simulink model "TMPC_3"  (Simulink 9.1)
settings: Solver=ode45  StartTime=0.0  StopTime=6  FixedStep=0.01  RelTol=1e-3  EnableMultiTasking=on
undefined symbols (not defined in the file): random_seeds
libraries: simulink x4, Solver_SF x1
settings Model: Creator=xuwei  LastModifiedBy=CK12
settings DataIOCC: LimitDataPoints=on
settings OptimizationCC: ExpressionDepthLimit=2147483647
settings DebuggingCC: SolverPrmCheckMsg=warning  FcnCallInpInsideContextMsg=warning  StateNameClashWarn=warning
settings ConfigComp: CovHtmlReporting=off

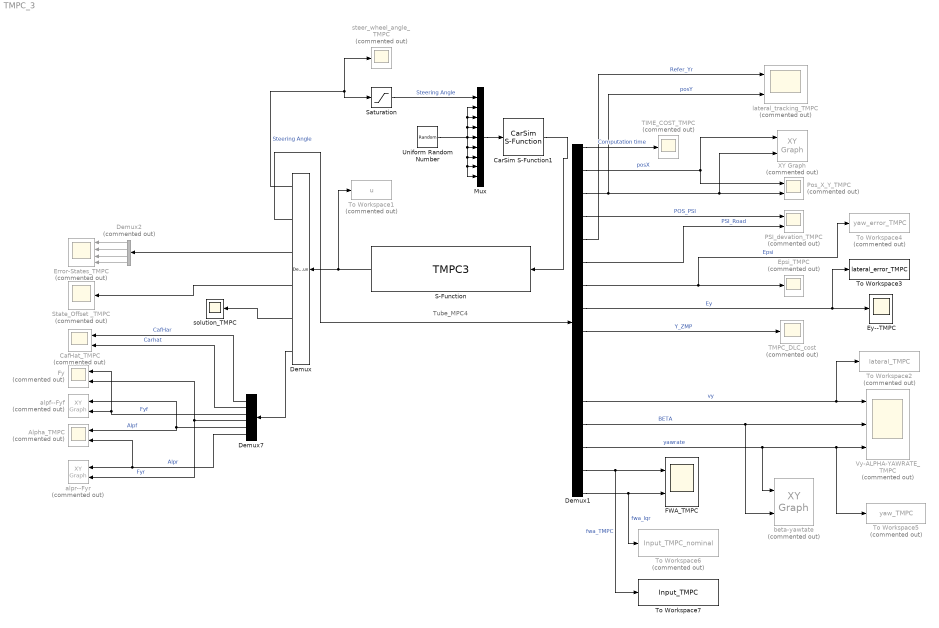
== system TMPC_3 ==
  note: Tube_MPC4
  Alpha_TMPC : Scope  Commented=on  NumInputPorts=2
  CafHat_TMPC : Scope  Commented=on  NumInputPorts=2
  CarSim S-Function1 : Solver_SF/CarSim S-Function  Priority=1  SIMFILE=simfile.sim  Run_RTs=off  vs_state_ind=Run  StopMode_ind=Vehicle Model
  Demux : Demux  Outputs=[1 16 4 4 1 6]
  Demux1 : Demux  Outputs=16
  Demux2 : Demux  Commented=on
  Demux7 : Demux  Outputs=6
  Epsi_TMPC : Scope  Commented=on
  Error-States_TMPC : Scope  Commented=on  NumInputPorts=4
  Ey--TMPC : Scope
  FWA_TMPC : Scope  NumInputPorts=2
  Fy : Scope  Commented=on  NumInputPorts=2
  Mux : Mux  Inputs=9
  PSI_devation_TMPC : Scope  Commented=on  NumInputPorts=2
  Pos_X_Y_TMPC : Scope  Commented=on  NumInputPorts=2
  S-Function : S-Function  FunctionName=TMPC3  SFunctionDeploymentMode=off  EnableBusSupport=off
  Saturation : Saturate  UpperLimit=430  LowerLimit=-430
  State_Offset _TMPC : Scope  Commented=on
  TIME_COST_TMPC : Scope  Commented=on
  TMPC_DLC_cost : Scope  Commented=on
  To Workspace1 : ToWorkspace  Commented=on  VariableName=u  SaveFormat=Structure  SampleTime=-1
  To Workspace2 : ToWorkspace  Commented=on  VariableName=lateral_TMPC  SaveFormat=Timeseries  SampleTime=-1
  To Workspace3 : ToWorkspace  VariableName=lateral_error_TMPC  SaveFormat=Timeseries  SampleTime=-1
  To Workspace4 : ToWorkspace  Commented=on  VariableName=yaw_error_TMPC  SaveFormat=Timeseries  SampleTime=-1
  To Workspace5 : ToWorkspace  Commented=on  VariableName=yaw_TMPC  SaveFormat=Timeseries  SampleTime=-1
  To Workspace6 : ToWorkspace  Commented=on  VariableName=Input_TMPC_nominal  SaveFormat=Timeseries  SampleTime=-1
  To Workspace7 : ToWorkspace  VariableName=Input_TMPC  SaveFormat=Timeseries  SampleTime=-1
  Uniform Random Number : UniformRandomNumber  Minimum=0.4  Maximum=0.8  Seed=random_seeds  SampleTime=0.1
  Vy-ALPHA-YAWRATE_TMPC : Scope  Commented=on  NumInputPorts=3
  XY Graph : simulink/Sinks/XY Graph  Commented=on  xmin=-10  xmax=180  ymin=-4  ymax=4  st=-1
  alpf--Fyf : simulink/Sinks/XY Graph  Commented=on  xmin=-0.15  xmax=0.15  ymin=-8000  ymax=8000  st=-1
  alpr--Fyr : simulink/Sinks/XY Graph  Commented=on  xmin=-0.1  xmax=0.1  ymin=-6000  ymax=6000  st=-1
  beta-yawtate : simulink/Sinks/XY Graph  Commented=on  xmin=-0.7  xmax=0.7  ymin=-0.1  ymax=0.1  st=-1
  lateral_tracking_TMPC : Scope  Commented=on  NumInputPorts=2
  "solution_TMPC " : Scope
  steer_wheel_angle_TMPC : Scope  Commented=on
  wires:
  CarSim S-Function1/1 -> S-Function/1
  S-Function/1 -> To Workspace1/1, Demux/1
  Demux/2 -> Demux1/1
  Demux2/1 -> Error-States_TMPC/1
  Demux2/2 -> Error-States_TMPC/2
  Demux2/3 -> Error-States_TMPC/3
  Demux2/4 -> Error-States_TMPC/4
  Demux/3 -> Demux2/1
  Demux1/6 -> PSI_devation_TMPC/2  "PSI_Road"
  Demux1/14 -> To Workspace5/1, Vy-ALPHA-YAWRATE_TMPC/3, beta-yawtate/1  "yawrate"
  Demux1/4 -> PSI_devation_TMPC/1  "POS_PSI"
  Demux1/9 -> TMPC_DLC_cost/1  "Y_ZMP"
  Demux1/12 -> Vy-ALPHA-YAWRATE_TMPC/1, To Workspace2/1  "vy"
  Demux1/5 -> lateral_tracking_TMPC/1  "Refer_Yr"
  Demux1/13 -> Vy-ALPHA-YAWRATE_TMPC/2, beta-yawtate/2  "BETA"
  Demux1/16 -> To Workspace6/1, FWA_TMPC/2  "fwa_lqr"
  Demux/5 -> "solution_TMPC "/1
  Demux/6 -> Demux7/1
  Demux7/1 -> CafHat_TMPC/1  "CafHar"
  Demux7/2 -> CafHat_TMPC/2  "Carhat"
  Demux7/3 -> Fy/1, alpf--Fyf/2  "Fyf"
  Demux7/4 -> Fy/2, alpr--Fyr/2  "Fyr"
  Demux7/5 -> alpf--Fyf/1, Alpha_TMPC/1  "Alpf"
  Demux7/6 -> alpr--Fyr/1, Alpha_TMPC/2  "Alpr"
  Demux1/3 -> XY Graph/2, Pos_X_Y_TMPC/2, lateral_tracking_TMPC/2  "posY"
  Demux1/1 -> TIME_COST_TMPC/1  "Computation time"
  Demux1/2 -> Pos_X_Y_TMPC/1, XY Graph/1  "posX"
  Demux1/7 -> Epsi_TMPC/1, To Workspace4/1  "Epsi"
  Demux/1 -> steer_wheel_angle_TMPC/1, Saturation/1  "Steering Angle"
  Demux1/8 -> Ey--TMPC/1, To Workspace3/1  "Ey"
  Demux1/15 -> To Workspace7/1, FWA_TMPC/1  "fwa_TMPC"
  Demux/4 -> State_Offset _TMPC/1
  Mux/1 -> CarSim S-Function1/1
  Uniform Random Number/1 -> Mux/9, Mux/8, Mux/7, Mux/6, Mux/5, Mux/2, Mux/3, Mux/4
  Saturation/1 -> Mux/1  "Steering Angle"
